simulink model "FitNormalDist"  (R2020b)
settings: Solver=VariableStepAuto  StartTime=0.0  StopTime=200  RelTol=1e-3
settings Model: Creator=yongjiaf  LastModifiedBy=yongjiaf

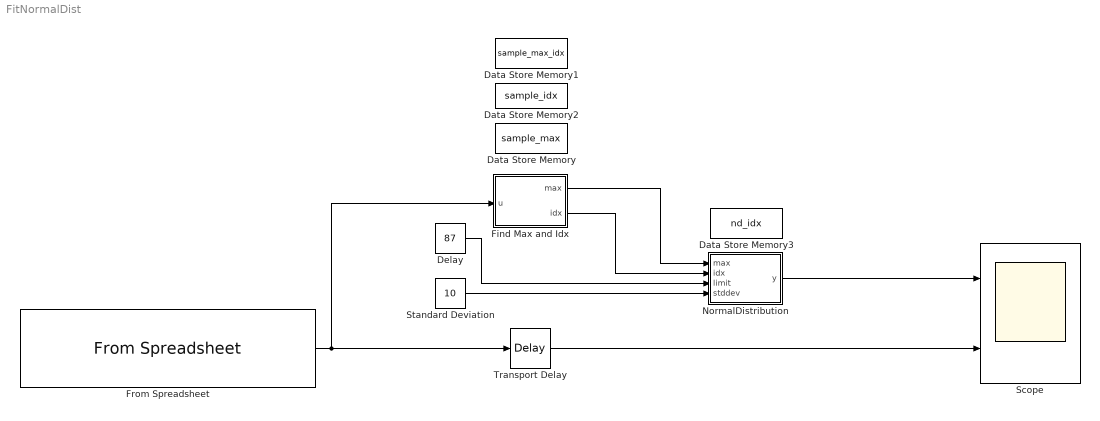
== system FitNormalDist ==
  Data Store Memory : DataStoreMemory  DataStoreName=sample_max  ReadBeforeWriteMsg=warning  WriteAfterWriteMsg=warning  WriteAfterReadMsg=warning  ShowAdditionalParam=off  OutDataTypeStr=double
  Data Store Memory1 : DataStoreMemory  DataStoreName=sample_max_idx  ReadBeforeWriteMsg=warning  WriteAfterWriteMsg=warning  WriteAfterReadMsg=warning  ShowAdditionalParam=off  OutDataTypeStr=uint32
  Data Store Memory2 : DataStoreMemory  DataStoreName=sample_idx  ReadBeforeWriteMsg=warning  WriteAfterWriteMsg=warning  WriteAfterReadMsg=warning  ShowAdditionalParam=off  OutDataTypeStr=uint32
  Data Store Memory3 : DataStoreMemory  DataStoreName=nd_idx  ReadBeforeWriteMsg=warning  WriteAfterWriteMsg=warning  WriteAfterReadMsg=warning  ShowAdditionalParam=off  OutDataTypeStr=uint32
  Delay : Constant  Value=87
  Find Max and Idx : MATLAB Function  TreatAsAtomicUnit=on
  From Spreadsheet : FromSpreadsheet  FileName=/home/yongjiaf/Desktop/UsefulScripts/MassData.xlsx  SheetName=MassData  Range=B2:B87  OutDataTypeStr=double  TreatFirstColumnAs=Data  SampleTime=1  OutputAfterLastPoint=Ground value
  NormalDistribution : MATLAB Function  TreatAsAtomicUnit=on
  Scope : Scope  NumInputPorts=2
  Standard Deviation : Constant  Value=10
  Transport Delay : TransportDelay  DelayTime=87
  wires:
  From Spreadsheet/1 -> Find Max and Idx/1(u), Transport Delay/1
  Find Max and Idx/1(max) -> NormalDistribution/1(max)
  Find Max and Idx/2(idx) -> NormalDistribution/2(idx)
  Standard Deviation/1 -> NormalDistribution/4(stddev)
  Transport Delay/1 -> Scope/2
  NormalDistribution/1(y) -> Scope/1
  Delay/1 -> NormalDistribution/3(limit)

== matlab function FitNormalDist/NormalDistribution ==
  data: max input; idx input; limit input; y output; stddev input; nd_idx data_store_memory
function y = fcn(max, idx, limit, stddev)
global nd_idx;
nd_idx = nd_idx + 1;
if nd_idx < limit
    y = 0.0;
else
    idxf = cast(idx, 'double');
    nidxf = cast((nd_idx - limit), 'double');
    nd = normpdf(nidxf, idxf, stddev);
    ndmax = normpdf(idxf, idxf, stddev);
    y = max*nd/ndmax;
end

== matlab function FitNormalDist/Find Max and Idx ==
  data: u input; max output; idx output; sample_max data_store_memory; sample_idx data_store_memory; sample_max_idx data_store_memory
function [max, idx] = fcn(u)
global sample_max;
global sample_max_idx;
global sample_idx;

sample_idx = sample_idx + 1;
if u > sample_max
    sample_max = u;
    sample_max_idx = sample_idx;
end

max = sample_max;
idx = sample_max_idx;
